simulink model "FullModelAddANN_Final_ANN_revised"  (R2024b)
settings: Solver=ode4  StartTime=0.0  StopTime=40  FixedStep=1e-5  RelTol=1e-3
values from neighbouring files (symbols this model uses):
  Dp = 2.506338228783948e3    (= 2506.33822878)    [FullModelAddANNm_Final.m]    (also in main_opal_ann_control.m)
  Dq = 1.033099625954584    (= 1.03309962595)    [FullModelAddANNm_Final.m]    (also in main_opal_ann_control.m)
  Kp = 0.006383815167581    (= 0.00638381516758)    [FullModelAddANNm_Final.m]    (also in main_opal_ann_control.m)
  Kq = 0.076670166944346    (= 0.0766701669443)    [FullModelAddANNm_Final.m]    (also in main_opal_ann_control.m)
undefined symbols (not defined in the file or in its folder): Filter, Ls, params
libraries: neural x88, spsCurrentMeasurementLib x6, spsParallelRLCBranchLib x6, spsIGBTDiodeLib x6, spsMeanLib x6, spsSeriesRLCBranchLib x6, simulink x4, spsVoltageMeasurementLib x4, spsVariableInductorLib x3, spsVariableResistorLib x3, spsDCVoltageSourceLib x1, spsThreePhaseSourceLib x1
(part 1 of 11)
settings Model: SimulationMode=accelerator  Creator=Admin  LastModifiedBy=ACER
settings DataIOCC: SaveOutput=off  DSMLogging=off  SaveTime=off  ReturnWorkspaceOutputs=off
settings OptimizationCC: EfficientMapNaN2IntZero=off  AccelVerboseBuild=on
settings DebuggingCC: SignalInfNanChecking=error  CheckMatrixSingularityMsg=error  UnconnectedInputMsg=warning  UnconnectedOutputMsg=warning  UnconnectedLineMsg=warning
settings HardwareCC: TargetBitPerPointer=64  TargetBitPerSizeT=64  TargetBitPerPtrDiffT=64  TargetLongLongMode=on  TargetIntDivRoundTo=Zero  TargetEndianess=LittleEndian  TargetWordSize=64  TargetHWDeviceType=MATLAB Host  ProdEqTarget=off
settings ModelReferenceCC: EnableRefExpFcnMdlSchedulingChecks=on
settings SFSimCC: CustomCodeUndefinedFunction=UseInterfaceOnly
settings RTWCC: GPUComputeCapability=3.5
settings CodeAppCC: MaxIdLength=128
settings GRTTargetCC: TargetLangStandard=C89/C90 (ANSI)  CombineOutputUpdateFcns=off  GRTInterface=on

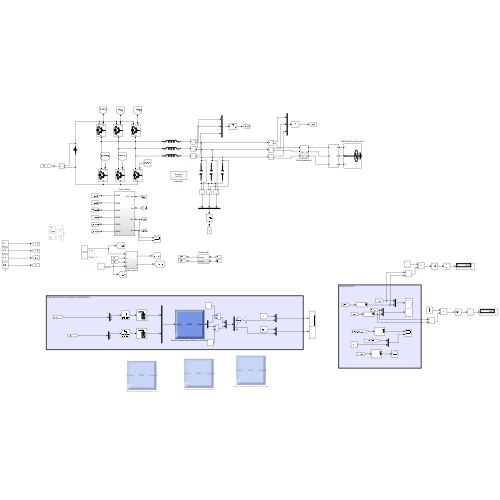
[thumbnail: Simulink's stored preview of the top-level diagram]
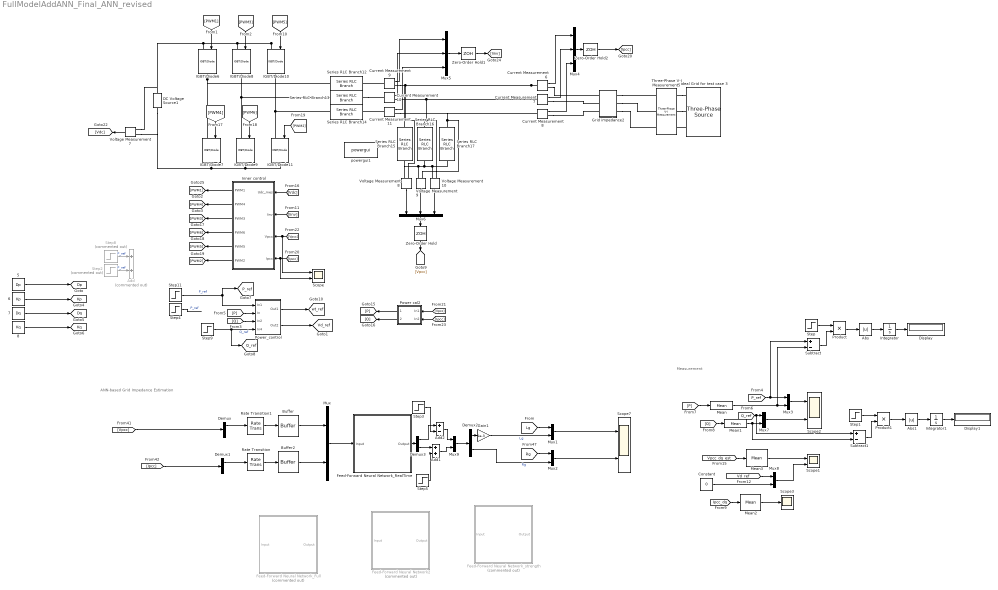
== system FullModelAddANN_Final_ANN_revised ==
  note: Measurement
  note: ANN-based Grid Impedance Estimation
  5 : Constant  Value=Dp
  6 : Constant  Value=Kp
  7 : Constant  Value=Dq
  8 : Constant  Value=Kq
  Abs : Abs  SaturateOnIntegerOverflow=off
  Abs1 : Abs  SaturateOnIntegerOverflow=off
  Add : Sum  Commented=on
  Add1 : Sum
  Add2 : Sum  Inputs=+-
  Buffer : Buffer  N=100  OutputFrames=off
  Buffer2 : Buffer  N=100  OutputFrames=off
  Constant : Constant  Value=0
  Current Measurement{6..11} (6 alike) : spsCurrentMeasurementLib/Current Measurement  PhasorSimulation=off  OutputType=Complex  PSBequivalent=0
  DC Voltage Source1 : spsDCVoltageSourceLib/DC Voltage Source  Amplitude=params.Vdc  Measurements=None
  Demux : Demux  Outputs=3
  Demux1 : Demux  Outputs=3
  Demux2 : Demux  Outputs=2
  Demux3 : Demux  Outputs=2
  Display : Display
  Display1 : Display
  Feed-Forward Neural Network2 : Subsystem  Commented=on
      mask help: Feed-Forward Neural Network
      mask Display: e = 0.06;c1 = [120 150 230]/255;c2 = ([120 150 230]+0)/383;c3 = ([120 150 230]+128)/383;patch([0 1 1 0],[0 0 1 1],c1);patch([0 1 1 1-e 1-e 0+e],[0 0 1 1-e 0+e 0+e],c2);patch([0 0 1 1-e 0+e 0+e],[0 1 1 1-e 1-e 0+e],c3);plot([0 1 1 0 0],[0 0 1 1 0]);fprintf('NNET');port_label('input',1,' Input');port_label('output',1,'Output ');
  Feed-Forward Neural Network_Full : Subsystem  Commented=on
      mask help: Feed-Forward Neural Network
      mask Display: e = 0.06;c1 = [120 150 230]/255;c2 = ([120 150 230]+0)/383;c3 = ([120 150 230]+128)/383;patch([0 1 1 0],[0 0 1 1],c1);patch([0 1 1 1-e 1-e 0+e],[0 0 1 1-e 0+e 0+e],c2);patch([0 0 1 1-e 0+e 0+e],[0 1 1 1-e 1-e 0+e],c3);plot([0 1 1 0 0],[0 0 1 1 0]);fprintf('NNET');port_label('input',1,' Input');port_label('output',1,'Output ');
  Feed-Forward Neural Network_RealTime : Subsystem
      mask help: Feed-Forward Neural Network
      mask Display: e = 0.06;c1 = [120 150 230]/255;c2 = ([120 150 230]+0)/383;c3 = ([120 150 230]+128)/383;patch([0 1 1 0],[0 0 1 1],c1);patch([0 1 1 1-e 1-e 0+e],[0 0 1 1-e 0+e 0+e],c2);patch([0 0 1 1-e 0+e 0+e],[0 1 1 1-e 1-e 0+e],c3);plot([0 1 1 0 0],[0 0 1 1 0]);fprintf('NNET');port_label('input',1,' Input');port_label('output',1,'Output ');
  Feed-Forward Neural Network_strength : Subsystem  Commented=on
      mask help: Feed-Forward Neural Network
      mask Display: e = 0.06;c1 = [120 150 230]/255;c2 = ([120 150 230]+0)/383;c3 = ([120 150 230]+128)/383;patch([0 1 1 0],[0 0 1 1],c1);patch([0 1 1 1-e 1-e 0+e],[0 0 1 1-e 0+e 0+e],c2);patch([0 0 1 1-e 0+e 0+e],[0 1 1 1-e 1-e 0+e],c3);plot([0 1 1 0 0],[0 0 1 1 0]);fprintf('NNET');port_label('input',1,' Input');port_label('output',1,'Output ');
  Gain1 : Gain  Gain=1e-3
  Grid impedance2 : Subsystem
  IGBT/Diode{6..11} (6 alike) : spsIGBTDiodeLib/IGBT//Diode  Ron=1e-3  Rs=1e5  Cs=inf  Measurements=off
  Ideal Grid for test case 3 : spsThreePhaseSourceLib/Three-Phase Source  InternalConnection=Yg  VoltagePhases=off  Voltage=params.Vj*sqrt(3)  PhaseAngle=0  Voltage_phases=[25e3 25e3 25e3]/sqrt(3)  PhaseAngles_phases=[0 -120 +120]  Frequency=params.f0  NonIdealSource=off  SpecifyImpedance=on  Resistance=0.8929  Inductance=16.58e-3  ShortCircuitLevel=params.SCR*params.S_rated  BaseVoltage=params.Vll_rms  XRratio=params.XR  BusType=swing  Pref=1e3  Qref=0  Prefabc=[10e3, 10e3, 10e3]  Qrefabc=[0, 0, 0]  Qmin=-inf  Qmax=inf
  Inner control : Subsystem
  Integrator : Integrator
  Integrator1 : Integrator
  Mean : spsMeanLib/Mean  Freq=50  Vinit=0  Ts=0
  Mean1 : spsMeanLib/Mean  Freq=50  Vinit=0  Ts=0
  Mean2 : spsMeanLib/Mean  Freq=60  Vinit=0  Ts=0
  Mean3 : spsMeanLib/Mean  Freq=60  Vinit=0  Ts=0
  Mux{,1..3,7..9} (7 alike) : Mux  Inputs=2
  Mux4 : Mux  Inputs=3
  Mux5 : Mux  Inputs=3
  Mux6 : Mux  Inputs=3
  Power cal2 : Subsystem
  Power_control : Subsystem
  Product : Product
  Product1 : Product
  Rate Transition : RateTransition  OutPortSampleTimeMultiple=2e-4  OutPortSampleTime=2e-4
  Rate Transition1 : RateTransition  OutPortSampleTimeMultiple=4  OutPortSampleTime=2e-4
  Scope{,1..2,7} (4 alike) : Scope  NumInputPorts=2
  Scope3 : Scope
  Series RLC Branch12 : spsSeriesRLCBranchLib/Series RLC Branch  LConnTagsString=__new0  RConnTagsString=__new0  BranchType=L  Resistance=Filter.Rs_1  Inductance=params.Filter.Ls_1  SetiL0=off  InitialCurrent=1  Capacitance=1e-6  Setx0=off  InitialVoltage=0  Measurements=None
  Series RLC Branch13 : spsSeriesRLCBranchLib/Series RLC Branch  LConnTagsString=__new0  RConnTagsString=__new0  BranchType=L  Resistance=Filter.Rs_1  Inductance=params.Filter.Ls_1  SetiL0=off  InitialCurrent=1  Capacitance=1e-6  Setx0=off  InitialVoltage=0  Measurements=None
  Series RLC Branch14 : spsSeriesRLCBranchLib/Series RLC Branch  LConnTagsString=__new0  RConnTagsString=__new0  BranchType=L  Resistance=Filter.Rs_1  Inductance=params.Filter.Ls_1  SetiL0=off  InitialCurrent=1  Capacitance=1e-6  Setx0=off  InitialVoltage=0  Measurements=None
  Series RLC Branch15 : spsSeriesRLCBranchLib/Series RLC Branch  LConnTagsString=__new0  RConnTagsString=__new0  BranchType=C  Resistance=1  Inductance=Ls  SetiL0=off  InitialCurrent=0  Capacitance=params.Filter.Cs  Setx0=off  InitialVoltage=0  Measurements=None
  Series RLC Branch16 : spsSeriesRLCBranchLib/Series RLC Branch  LConnTagsString=__new0  RConnTagsString=__new0  BranchType=C  Resistance=1  Inductance=Ls  SetiL0=off  InitialCurrent=0  Capacitance=params.Filter.Cs  Setx0=off  InitialVoltage=0  Measurements=None
  Series RLC Branch17 : spsSeriesRLCBranchLib/Series RLC Branch  LConnTagsString=__new0  RConnTagsString=__new0  BranchType=C  Resistance=1  Inductance=Ls  SetiL0=off  InitialCurrent=0  Capacitance=params.Filter.Cs  Setx0=off  InitialVoltage=0  Measurements=None
  Step : Step  Time=20  SampleTime=0
  Step1 : Step  Time=20  SampleTime=0
  Step11 : Step  Time=30  Before=3.5e3  After=4e3  SampleTime=0
  Step2 : Step  Commented=on  Time=70  After=0.5e3  SampleTime=0
  Step3 : Step  Time=20  After=4.08  SampleTime=0
  Step4 : Step  Time=70  After=0.5e3  SampleTime=0
  Step5 : Step  Time=20  SampleTime=0
  Step8 : Step  Commented=on  Time=50  Before=4e3  After=3.5e3  SampleTime=0
  Step9 : Step  Time=90  Before=params.Qref  After=params.Qref-0.5e3  SampleTime=0
  Subtract : Sum  Inputs=+-
  Subtract1 : Sum  Inputs=+-
  Three-Phase V-I Measurement5 : spsThreePhaseVIMeasurementLib/Three-Phase V-I Measurement  VoltageMeasurement=no  SetLabelV=off  LabelV=Vabc  Vpu=off  VpuLL=off  CurrentMeasurement=no  SetLabelI=off  LabelI=Iabc  Ipu=off  Pbase=100e6  Vbase=500e3  OutputType=Complex  PhasorSimulation=off  PSBequivalent=0
  Voltage Measurement{7..10} (4 alike) : spsVoltageMeasurementLib/Voltage Measurement  PhasorSimulation=off  OutputType=Complex  PSBequivalent=0
  Zero-Order Hold : ZeroOrderHold  SampleTime=5e-5
  Zero-Order Hold1 : ZeroOrderHold  SampleTime=5e-5
  Zero-Order Hold2 : ZeroOrderHold  SampleTime=5e-5
  powergui1 : sps_lib/powergui  Priority=1  SimulationMode=Discrete  SampleTime=1e-5  frequency=60  Iterations=50  frequencyindice=0  Pbase=100e6  ErrMax=1e-4  UnitsV=kV  UnitsW=MW  buscounter=0  FunctionMessages=off  echomessages=off  EnableUseOfTLC=off  CurrentSourceSwitches=off  DisableSnubberDevices=off  DisableRonSwitches=off  DisableVfSwitches=off  DisplayEquations=off  AutomaticDiscreteSolvers=on  SolverType=Tustin/Backward Euler (TBE)  Interpol=off  ExternalGateDelay=off  methode=off  Ts=100  x0status=blocks  SPID=on  SwTol=0  HookPort=off  NonlinearTolerance=0  nMaxIteration=15  ContinueOnMaxIteration=off  RestoreLinks=warning  ResistiveCurrentMeasurement=off  Frange=[0:2:500]  Ylog=off  Xlog=on  ShowGrid=off  save=off  variable=ZData  structure=0  ZoomFFT=off  StartTime=0.0  cycles=1  DisplayStyle=1  fundamental=60  FreqAxis=off  MaxFrequency=1000  frequencyindicesteady=1  RmsSteady=1  display=off
  tag scope: Dp=global, Dq=global, Kp=global, Kq=global, P_ref=global, Q_ref=global, Vd_ref=global, wt_ref=global
  wires:
  Step8/1 -> Add/1  "P_ref"
  Step2/1 -> Add/2  "P_ref"
  [Iinv] -> Inner control/2(Iinv)
  Inner control/1(PWM1) -> [PWM1]
  Inner control/4("PWM6 ") -> [PWM6]
  Inner control/6(PWM2) -> [PWM2]
  Voltage Measurement7/1 -> [Vdc]
  Inner control/5(PWM5) -> [PWM5]
  Voltage Measurement9/1 -> Mux6/2
  Mux5/1 -> Zero-Order Hold1/1
  [PWM6] -> IGBT/Diode9/1
  [PWM1] -> IGBT/Diode6/1
  [Ipcc] -> Scope/2, Inner control/4(Ipcc)
  [Vdc] -> Inner control/1(Udc_mes)
  [Vpcc] -> Scope/1, Inner control/3(Vpcc)
  Inner control/3(PWM3) -> [PWM3]
  Inner control/2("PWM4 ") -> [PWM4]
  Current Measurement11/1 -> Mux5/3
  Voltage Measurement10/1 -> Mux6/3
  [PWM2] -> IGBT/Diode11/1
  Mux4/1 -> Zero-Order Hold2/1
  [PWM4] -> IGBT/Diode7/1
  Mux6/1 -> Zero-Order Hold/1
  [PWM5] -> IGBT/Diode10/1
  Current Measurement8/1 -> Mux4/3
  Voltage Measurement8/1 -> Mux6/1
  Current Measurement9/1 -> Mux5/1
  Current Measurement7/1 -> Mux4/2
  Current Measurement6/1 -> Mux4/1
  Current Measurement10/1 -> Mux5/2
  [PWM3] -> IGBT/Diode8/1
  Power cal2/2(deltay2) -> [Q]
  Power cal2/1(deltay1) -> [P]
  [Vpcc] -> Power cal2/1(In1)
  [Ipcc] -> Power cal2/2(In2)
  Zero-Order Hold/1 -> [Vpcc]
  Zero-Order Hold1/1 -> [Iinv]
  Zero-Order Hold2/1 -> [Ipcc]
  5/1 -> [Dp]
  6/1 -> [Kp]
  7/1 -> [Dq]
  8/1 -> [Kq]
  Rate Transition1/1 -> Buffer/1
  Demux1/1 -> Rate Transition/1
  Demux/1 -> Rate Transition1/1
  Rate Transition/1 -> Buffer2/1
  Buffer2/1 -> Mux/2
  Buffer/1 -> Mux/1
  Mux/1 -> Feed-Forward Neural Network_RealTime/1(Input)
  Demux2/1 -> Gain1/1
  [P] -> Power_control/2(In)
  [Q] -> Power_control/3(In2)
  Power_control/1(Out1) -> [wt_ref]
  Power_control/2(Out2) -> [Vd_ref]
  [Lg] -> Mux1/1
  Gain1/1 -> Mux1/2  "Lg"
  [Rg] -> Mux2/1
  Demux2/2 -> Mux2/2  "Rg"
  Mux1/1 -> Scope7/1
  Mux2/1 -> Scope7/2
  [Vpcc] -> Demux/1
  [Ipcc] -> Demux1/1
  [Q] -> Mean1/1
  [P] -> Mean/1
  [Q_ref] -> Subtract1/1, Mux7/1
  Mux7/1 -> Scope2/2
  [P_ref] -> Subtract/1, Mux3/1
  Mux3/1 -> Scope2/1
  Mean1/1 -> Subtract1/2, Mux7/2
  Mean/1 -> Subtract/2, Mux3/2
  Mux8/1 -> Scope1/2
  Mean2/1 -> Scope3/1
  Constant/1 -> Mux8/2
  Mean3/1 -> Scope1/1
  [Vpcc_dq_est] -> Mean3/1
  [Ipcc_dq] -> Mean2/1
  [Vd_ref] -> Mux8/1
  Step4/1 -> ?  "P_ref"
  Step11/1 -> Power_control/1(In1), [P_ref]  "P_ref"
  Step9/1 -> [Q_ref], Power_control/4(In4)  "Q_ref"
  Abs/1 -> Integrator/1
  Integrator/1 -> Display/1
  Integrator1/1 -> Display1/1
  Abs1/1 -> Integrator1/1
  Step/1 -> Product/1
  Subtract/1 -> Product/2
  Product/1 -> Abs/1
  Step1/1 -> Product1/1
  Subtract1/1 -> Product1/2
  Product1/1 -> Abs1/1
  Feed-Forward Neural Network_RealTime/1(Output) -> Demux3/1
  Mux9/1 -> Demux2/1
  Demux3/1 -> Add2/1
  Add2/1 -> Mux9/1
  Demux3/2 -> Add1/1
  Add1/1 -> Mux9/2
  Step5/1 -> Add1/2
  Step3/1 -> Add2/2
  connections:
  Series RLC Branch14/LConn1 -- IGBT/Diode10/RConn1 -- IGBT/Diode11/LConn1
  Series RLC Branch17/LConn1 -- Current Measurement11/RConn1 -- Current Measurement8/LConn1 -- Voltage Measurement10/LConn1
  IGBT/Diode6/RConn1 -- Series RLC Branch12/LConn1 -- IGBT/Diode7/LConn1
  Voltage Measurement10/LConn2 -- Series RLC Branch17/RConn1 -- Voltage Measurement8/LConn2 -- Series RLC Branch15/RConn1 -- Voltage Measurement9/LConn2 -- Series RLC Branch16/RConn1
  Current Measurement6/LConn1 -- Series RLC Branch15/LConn1 -- Voltage Measurement8/LConn1 -- Current Measurement9/RConn1
  IGBT/Diode10/LConn1 -- DC Voltage Source1/RConn1 -- Voltage Measurement7/LConn1 -- IGBT/Diode6/LConn1 -- IGBT/Diode8/LConn1
  IGBT/Diode7/RConn1 -- IGBT/Diode11/RConn1 -- IGBT/Diode9/RConn1 -- Voltage Measurement7/LConn2 -- DC Voltage Source1/LConn1
  Series RLC Branch13/LConn1 -- IGBT/Diode8/RConn1 -- IGBT/Diode9/LConn1
  Current Measurement7/LConn1 -- Current Measurement10/RConn1 -- Series RLC Branch16/LConn1 -- Voltage Measurement9/LConn1
  Current Measurement7/RConn1 -- Grid impedance2/LConn2
  Current Measurement11/LConn1 -- Series RLC Branch14/RConn1
  Current Measurement8/RConn1 -- Grid impedance2/LConn3
  Series RLC Branch13/RConn1 -- Current Measurement10/LConn1
  Current Measurement9/LConn1 -- Series RLC Branch12/RConn1
  Current Measurement6/RConn1 -- Grid impedance2/LConn1
  Grid impedance2/RConn1 -- Three-Phase V-I Measurement5/RConn3
  Three-Phase V-I Measurement5/LConn2 -- Ideal Grid for test case 3/RConn2
  Three-Phase V-I Measurement5/LConn3 -- Ideal Grid for test case 3/RConn3
  Grid impedance2/RConn2 -- Three-Phase V-I Measurement5/RConn2
  Ideal Grid for test case 3/RConn1 -- Three-Phase V-I Measurement5/LConn1
  Grid impedance2/RConn3 -- Three-Phase V-I Measurement5/RConn1

== system FullModelAddANN_Final_ANN_revised/Feed-Forward Neural Network2 ==
  Input : Inport  PortDimensions=200
      mask Display: e = 0.06;c1 = [120 230 180]/255;c2 = ([120 230 180]+0)/(256+128);c3 = ([120 230 180]+128)/(256+128);patch([0 1 1 0],[0 0 1 1],c1);patch([0 1 1 1-e 1-e 0+e],[0 0 1 1-e 0+e 0+e],c2);patch([0 0 1 1-e 0+e 0+e],[0 1 1 1-e 1-e 0+e],c3);plot([0 1 1 0 0],[0 0 1 1 0]);
  Layer 1 : Subsystem
      mask Display: e = 0.06;c1 = [120 150 230]/255;c2 = ([120 150 230]+0)/383;c3 = ([120 150 230]+128)/383;patch([0 1 1 0],[0 0 1 1],c1);patch([0 1 1 1-e 1-e 0+e],[0 0 1 1-e 0+e 0+e],c2);patch([0 0 1 1-e 0+e 0+e],[0 1 1 1-e 1-e 0+e],c3);plot([0 1 1 0 0],[0 0 1 1 0]);
  Layer 2 : Subsystem
      mask Display: e = 0.06;c1 = [120 150 230]/255;c2 = ([120 150 230]+0)/383;c3 = ([120 150 230]+128)/383;patch([0 1 1 0],[0 0 1 1],c1);patch([0 1 1 1-e 1-e 0+e],[0 0 1 1-e 0+e 0+e],c2);patch([0 0 1 1-e 0+e 0+e],[0 1 1 1-e 1-e 0+e],c3);plot([0 1 1 0 0],[0 0 1 1 0]);
  Process Input 1 : Subsystem
      mask Display: e = 0.06;c1 = [120 150 230]/255;c2 = ([120 150 230]+0)/383;c3 = ([120 150 230]+128)/383;patch([0 1 1 0],[0 0 1 1],c1);patch([0 1 1 1-e 1-e 0+e],[0 0 1 1-e 0+e 0+e],c2);patch([0 0 1 1-e 0+e 0+e],[0 1 1 1-e 1-e 0+e],c3);plot([0 1 1 0 0],[0 0 1 1 0]);
  Process Output 1 : Subsystem
      mask Display: e = 0.06;c1 = [120 150 230]/255;c2 = ([120 150 230]+0)/383;c3 = ([120 150 230]+128)/383;patch([0 1 1 0],[0 0 1 1],c1);patch([0 1 1 1-e 1-e 0+e],[0 0 1 1-e 0+e 0+e],c2);patch([0 0 1 1-e 0+e 0+e],[0 1 1 1-e 1-e 0+e],c3);plot([0 1 1 0 0],[0 0 1 1 0]);
  Output : Outport  InitialOutput=[0;0]
      mask Display: e = 0.06;c1 = [120 230 180]/255;c2 = ([120 230 180]+0)/(256+128);c3 = ([120 230 180]+128)/(256+128);patch([0 1 1 0],[0 0 1 1],c1);patch([0 1 1 1-e 1-e 0+e],[0 0 1 1-e 0+e 0+e],c2);patch([0 0 1 1-e 0+e 0+e],[0 1 1 1-e 1-e 0+e],c3);plot([0 1 1 0 0],[0 0 1 1 0]);
  wires:
  Input/1 -> Process Input 1/1(x)
  Process Output 1/1(y) -> Output/1
  Process Input 1/1(p) -> Layer 1/1("p{1}")
  Layer 1/1("a{1}") -> [feedback1]
  [feedback1] -> Layer 2/1("a{1} ")
  Layer 2/1("a{2}") -> Process Output 1/1(a)

== system FullModelAddANN_Final_ANN_revised/Feed-Forward Neural Network_Full ==
  Input : Inport  PortDimensions=200
      mask Display: e = 0.06;c1 = [120 230 180]/255;c2 = ([120 230 180]+0)/(256+128);c3 = ([120 230 180]+128)/(256+128);patch([0 1 1 0],[0 0 1 1],c1);patch([0 1 1 1-e 1-e 0+e],[0 0 1 1-e 0+e 0+e],c2);patch([0 0 1 1-e 0+e 0+e],[0 1 1 1-e 1-e 0+e],c3);plot([0 1 1 0 0],[0 0 1 1 0]);
  Layer 1 : Subsystem
      mask Display: e = 0.06;c1 = [120 150 230]/255;c2 = ([120 150 230]+0)/383;c3 = ([120 150 230]+128)/383;patch([0 1 1 0],[0 0 1 1],c1);patch([0 1 1 1-e 1-e 0+e],[0 0 1 1-e 0+e 0+e],c2);patch([0 0 1 1-e 0+e 0+e],[0 1 1 1-e 1-e 0+e],c3);plot([0 1 1 0 0],[0 0 1 1 0]);
  Layer 2 : Subsystem
      mask Display: e = 0.06;c1 = [120 150 230]/255;c2 = ([120 150 230]+0)/383;c3 = ([120 150 230]+128)/383;patch([0 1 1 0],[0 0 1 1],c1);patch([0 1 1 1-e 1-e 0+e],[0 0 1 1-e 0+e 0+e],c2);patch([0 0 1 1-e 0+e 0+e],[0 1 1 1-e 1-e 0+e],c3);plot([0 1 1 0 0],[0 0 1 1 0]);
  Process Input 1 : Subsystem
      mask Display: e = 0.06;c1 = [120 150 230]/255;c2 = ([120 150 230]+0)/383;c3 = ([120 150 230]+128)/383;patch([0 1 1 0],[0 0 1 1],c1);patch([0 1 1 1-e 1-e 0+e],[0 0 1 1-e 0+e 0+e],c2);patch([0 0 1 1-e 0+e 0+e],[0 1 1 1-e 1-e 0+e],c3);plot([0 1 1 0 0],[0 0 1 1 0]);
  Process Output 1 : Subsystem
      mask Display: e = 0.06;c1 = [120 150 230]/255;c2 = ([120 150 230]+0)/383;c3 = ([120 150 230]+128)/383;patch([0 1 1 0],[0 0 1 1],c1);patch([0 1 1 1-e 1-e 0+e],[0 0 1 1-e 0+e 0+e],c2);patch([0 0 1 1-e 0+e 0+e],[0 1 1 1-e 1-e 0+e],c3);plot([0 1 1 0 0],[0 0 1 1 0]);
  Output : Outport  InitialOutput=[0;0]
      mask Display: e = 0.06;c1 = [120 230 180]/255;c2 = ([120 230 180]+0)/(256+128);c3 = ([120 230 180]+128)/(256+128);patch([0 1 1 0],[0 0 1 1],c1);patch([0 1 1 1-e 1-e 0+e],[0 0 1 1-e 0+e 0+e],c2);patch([0 0 1 1-e 0+e 0+e],[0 1 1 1-e 1-e 0+e],c3);plot([0 1 1 0 0],[0 0 1 1 0]);
  wires:
  Input/1 -> Process Input 1/1(x)
  Process Output 1/1(y) -> Output/1
  Process Input 1/1(p) -> Layer 1/1("p{1}")
  Layer 1/1("a{1}") -> [feedback1]
  [feedback1] -> Layer 2/1("a{1} ")
  Layer 2/1("a{2}") -> Process Output 1/1(a)

== system FullModelAddANN_Final_ANN_revised/Feed-Forward Neural Network_RealTime ==
  Input : Inport  PortDimensions=200
      mask Display: e = 0.06;c1 = [120 230 180]/255;c2 = ([120 230 180]+0)/(256+128);c3 = ([120 230 180]+128)/(256+128);patch([0 1 1 0],[0 0 1 1],c1);patch([0 1 1 1-e 1-e 0+e],[0 0 1 1-e 0+e 0+e],c2);patch([0 0 1 1-e 0+e 0+e],[0 1 1 1-e 1-e 0+e],c3);plot([0 1 1 0 0],[0 0 1 1 0]);
  Layer 1 : Subsystem
      mask Display: e = 0.06;c1 = [120 150 230]/255;c2 = ([120 150 230]+0)/383;c3 = ([120 150 230]+128)/383;patch([0 1 1 0],[0 0 1 1],c1);patch([0 1 1 1-e 1-e 0+e],[0 0 1 1-e 0+e 0+e],c2);patch([0 0 1 1-e 0+e 0+e],[0 1 1 1-e 1-e 0+e],c3);plot([0 1 1 0 0],[0 0 1 1 0]);
  Layer 2 : Subsystem
      mask Display: e = 0.06;c1 = [120 150 230]/255;c2 = ([120 150 230]+0)/383;c3 = ([120 150 230]+128)/383;patch([0 1 1 0],[0 0 1 1],c1);patch([0 1 1 1-e 1-e 0+e],[0 0 1 1-e 0+e 0+e],c2);patch([0 0 1 1-e 0+e 0+e],[0 1 1 1-e 1-e 0+e],c3);plot([0 1 1 0 0],[0 0 1 1 0]);
  Process Input 1 : Subsystem
      mask Display: e = 0.06;c1 = [120 150 230]/255;c2 = ([120 150 230]+0)/383;c3 = ([120 150 230]+128)/383;patch([0 1 1 0],[0 0 1 1],c1);patch([0 1 1 1-e 1-e 0+e],[0 0 1 1-e 0+e 0+e],c2);patch([0 0 1 1-e 0+e 0+e],[0 1 1 1-e 1-e 0+e],c3);plot([0 1 1 0 0],[0 0 1 1 0]);
  Process Output 1 : Subsystem
      mask Display: e = 0.06;c1 = [120 150 230]/255;c2 = ([120 150 230]+0)/383;c3 = ([120 150 230]+128)/383;patch([0 1 1 0],[0 0 1 1],c1);patch([0 1 1 1-e 1-e 0+e],[0 0 1 1-e 0+e 0+e],c2);patch([0 0 1 1-e 0+e 0+e],[0 1 1 1-e 1-e 0+e],c3);plot([0 1 1 0 0],[0 0 1 1 0]);
  Output : Outport  InitialOutput=[0;0]
      mask Display: e = 0.06;c1 = [120 230 180]/255;c2 = ([120 230 180]+0)/(256+128);c3 = ([120 230 180]+128)/(256+128);patch([0 1 1 0],[0 0 1 1],c1);patch([0 1 1 1-e 1-e 0+e],[0 0 1 1-e 0+e 0+e],c2);patch([0 0 1 1-e 0+e 0+e],[0 1 1 1-e 1-e 0+e],c3);plot([0 1 1 0 0],[0 0 1 1 0]);
  wires:
  Input/1 -> Process Input 1/1(x)
  Process Output 1/1(y) -> Output/1
  Process Input 1/1(p) -> Layer 1/1("p{1}")
  Layer 1/1("a{1}") -> [feedback1]
  [feedback1] -> Layer 2/1("a{1} ")
  Layer 2/1("a{2}") -> Process Output 1/1(a)

== system FullModelAddANN_Final_ANN_revised/Feed-Forward Neural Network_strength ==
  Input : Inport  PortDimensions=200
      mask Display: e = 0.06;c1 = [120 230 180]/255;c2 = ([120 230 180]+0)/(256+128);c3 = ([120 230 180]+128)/(256+128);patch([0 1 1 0],[0 0 1 1],c1);patch([0 1 1 1-e 1-e 0+e],[0 0 1 1-e 0+e 0+e],c2);patch([0 0 1 1-e 0+e 0+e],[0 1 1 1-e 1-e 0+e],c3);plot([0 1 1 0 0],[0 0 1 1 0]);
  Layer 1 : Subsystem
      mask Display: e = 0.06;c1 = [120 150 230]/255;c2 = ([120 150 230]+0)/383;c3 = ([120 150 230]+128)/383;patch([0 1 1 0],[0 0 1 1],c1);patch([0 1 1 1-e 1-e 0+e],[0 0 1 1-e 0+e 0+e],c2);patch([0 0 1 1-e 0+e 0+e],[0 1 1 1-e 1-e 0+e],c3);plot([0 1 1 0 0],[0 0 1 1 0]);
  Layer 2 : Subsystem
      mask Display: e = 0.06;c1 = [120 150 230]/255;c2 = ([120 150 230]+0)/383;c3 = ([120 150 230]+128)/383;patch([0 1 1 0],[0 0 1 1],c1);patch([0 1 1 1-e 1-e 0+e],[0 0 1 1-e 0+e 0+e],c2);patch([0 0 1 1-e 0+e 0+e],[0 1 1 1-e 1-e 0+e],c3);plot([0 1 1 0 0],[0 0 1 1 0]);
  Process Input 1 : Subsystem
      mask Display: e = 0.06;c1 = [120 150 230]/255;c2 = ([120 150 230]+0)/383;c3 = ([120 150 230]+128)/383;patch([0 1 1 0],[0 0 1 1],c1);patch([0 1 1 1-e 1-e 0+e],[0 0 1 1-e 0+e 0+e],c2);patch([0 0 1 1-e 0+e 0+e],[0 1 1 1-e 1-e 0+e],c3);plot([0 1 1 0 0],[0 0 1 1 0]);
  Process Output 1 : Subsystem
      mask Display: e = 0.06;c1 = [120 150 230]/255;c2 = ([120 150 230]+0)/383;c3 = ([120 150 230]+128)/383;patch([0 1 1 0],[0 0 1 1],c1);patch([0 1 1 1-e 1-e 0+e],[0 0 1 1-e 0+e 0+e],c2);patch([0 0 1 1-e 0+e 0+e],[0 1 1 1-e 1-e 0+e],c3);plot([0 1 1 0 0],[0 0 1 1 0]);
  Output : Outport  InitialOutput=[0;0]
      mask Display: e = 0.06;c1 = [120 230 180]/255;c2 = ([120 230 180]+0)/(256+128);c3 = ([120 230 180]+128)/(256+128);patch([0 1 1 0],[0 0 1 1],c1);patch([0 1 1 1-e 1-e 0+e],[0 0 1 1-e 0+e 0+e],c2);patch([0 0 1 1-e 0+e 0+e],[0 1 1 1-e 1-e 0+e],c3);plot([0 1 1 0 0],[0 0 1 1 0]);
  wires:
  Input/1 -> Process Input 1/1(x)
  Process Output 1/1(y) -> Output/1
  Process Input 1/1(p) -> Layer 1/1("p{1}")
  Layer 1/1("a{1}") -> [feedback1]
  [feedback1] -> Layer 2/1("a{1} ")
  Layer 2/1("a{2}") -> Process Output 1/1(a)

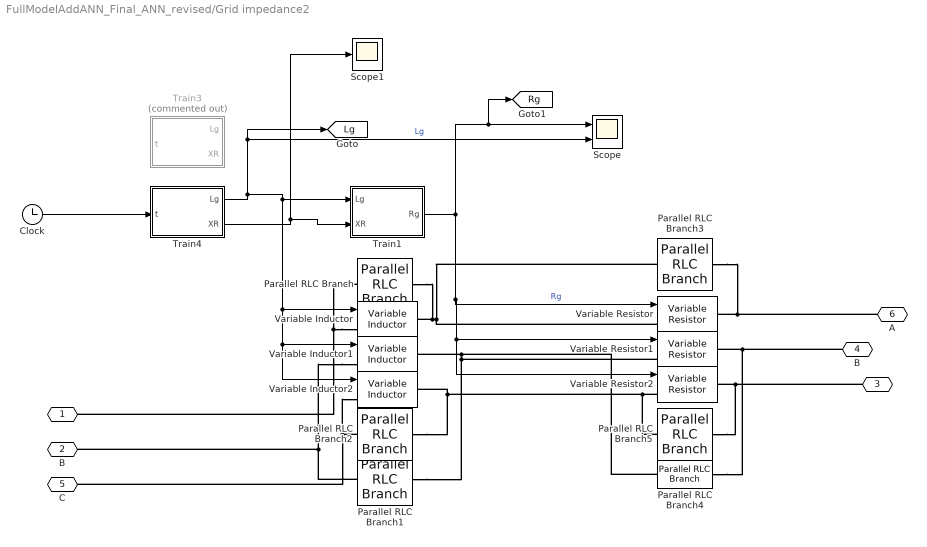
== system FullModelAddANN_Final_ANN_revised/Grid impedance2 ==
  Clock : Clock
      settings: Decimation=150
  Parallel RLC Branch{,1..5} (6 alike) : spsParallelRLCBranchLib/Parallel RLC Branch  LConnTagsString=a  RConnTagsString=__new0  BranchType=R  Resistance=1e6  Inductance=1e-3  SetiL0=off  InitialCurrent=0  Capacitance=1e-6  Setx0=off  InitialVoltage=0  Measurements=None
  Scope : Scope  NumInputPorts=2
  Scope1 : Scope
  Train1 : MATLAB Function  TreatAsAtomicUnit=on
  Train3 : MATLAB Function  Commented=on  TreatAsAtomicUnit=on
  Train4 : MATLAB Function  TreatAsAtomicUnit=on
  Variable Inductor : spsVariableInductorLib/Variable Inductor  methode=Backward Euler  Labsmin=1e-6  Initialize=off  iL0=0  L0=1e-3  Vl0=-0.0024759
  Variable Inductor1 : spsVariableInductorLib/Variable Inductor  methode=Backward Euler  Labsmin=1e-6  Initialize=off  iL0=0  L0=1e-3  Vl0=67.3622
  Variable Inductor2 : spsVariableInductorLib/Variable Inductor  methode=Backward Euler  Labsmin=1e-6  Initialize=off  iL0=0  L0=1e-3  Vl0=-67.3597
  Variable Resistor : spsVariableResistorLib/Variable Resistor  Rabsmin=1e-3
  Variable Resistor1 : spsVariableResistorLib/Variable Resistor  Rabsmin=1e-3
  Variable Resistor2 : spsVariableResistorLib/Variable Resistor  Rabsmin=1e-3
  "   " : PMIOPort  Side=Left
  "   B" : PMIOPort  Port=2  Side=Left
  "  " : PMIOPort  Port=3  Side=Right
  "  B" : PMIOPort  Port=4  Side=Right
  "   C" : PMIOPort  Port=5  Side=Left
  "  A" : PMIOPort  Port=6  Side=Right
  tag scope: Lg=global, Rg=global
  wires:
  Train1/1(Rg) -> Scope/1, [Rg], Variable Resistor/1, Variable Resistor1/1, Variable Resistor2/1  "Rg"
  Clock/1 -> Train4/1(t)
  Train4/1(Lg) -> [Lg], Scope/2, Variable Inductor/1, Variable Inductor1/1, Variable Inductor2/1, Train1/1(Lg)  "Lg"
  Train4/2(XR) -> Train1/2(XR), Scope1/1
  connections:
  Variable Resistor1/LConn1 -- Variable Inductor1/RConn1 -- Parallel RLC Branch4/LConn1 -- Parallel RLC Branch1/RConn1
  Variable Resistor2/LConn1 -- Parallel RLC Branch5/LConn1 -- Variable Inductor2/RConn1 -- Parallel RLC Branch2/RConn1
  Variable Resistor1/RConn1 -- Parallel RLC Branch4/RConn1 -- "  B"/RConn1
  Variable Resistor2/RConn1 -- Parallel RLC Branch5/RConn1 -- "  "/RConn1
  Variable Resistor/RConn1 -- Parallel RLC Branch3/RConn1 -- "  A"/RConn1
  Variable Inductor/LConn1 -- "   "/RConn1 -- Parallel RLC Branch/LConn1
  Variable Inductor/RConn1 -- Parallel RLC Branch3/LConn1 -- Variable Resistor/LConn1 -- Parallel RLC Branch/RConn1
  Variable Inductor1/LConn1 -- "   B"/RConn1 -- Parallel RLC Branch1/LConn1
  Variable Inductor2/LConn1 -- "   C"/RConn1 -- Parallel RLC Branch2/LConn1

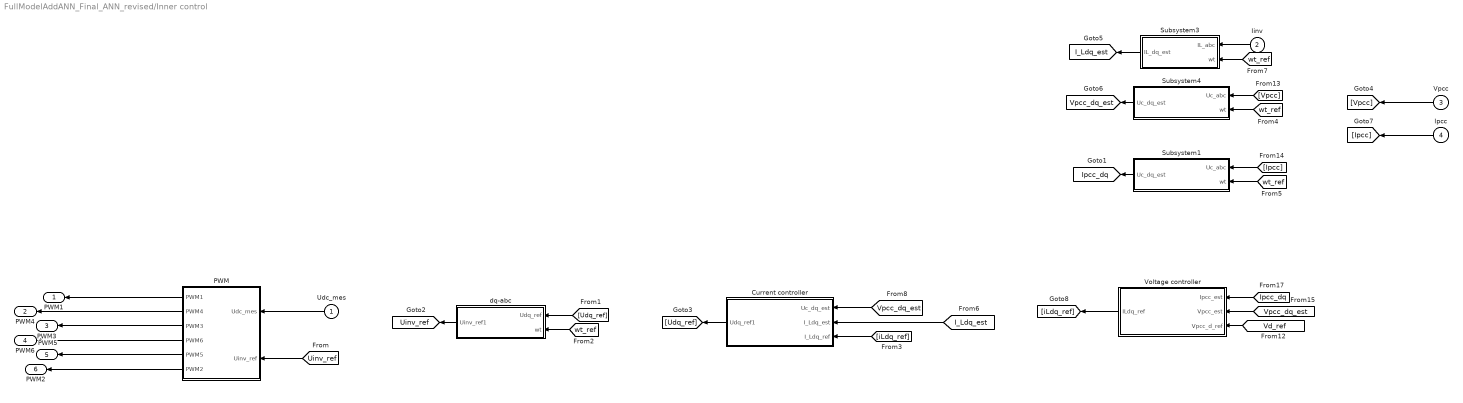
== system FullModelAddANN_Final_ANN_revised/Inner control ==
  Udc_mes : Inport
  Iinv : Inport  Port=2
  Vpcc : Inport  Port=3
  Ipcc : Inport  Port=4
  Current controller : Subsystem
  PWM : Subsystem
  Subsystem1 : Subsystem
  Subsystem3 : Subsystem
  Subsystem4 : Subsystem
  Voltage controller : Subsystem
  dq-abc : Subsystem
  PWM1 : Outport
  "PWM4 " : Outport  Port=2
  PWM3 : Outport  Port=3
  "PWM6 " : Outport  Port=4
  PWM5 : Outport  Port=5
  PWM2 : Outport  Port=6
  tag scope: I_Ldq_est=global, Ipcc_dq=global, Uinv_ref=global, Vpcc_dq_est=global
  wires:
  [Vpcc_dq_est] -> Current controller/1(Uc_dq_est)
  PWM/4("PWM6 ") -> "PWM6 "/1
  Udc_mes/1 -> PWM/1(Udc_mes)
  [I_Ldq_est] -> Current controller/2(I_Ldq_est)
  Subsystem4/1(Uc_dq_est) -> [Vpcc_dq_est]
  Current controller/1(Udq_ref1) -> [Udq_ref]
  [wt_ref] -> Subsystem3/2(wt)
  dq-abc/1(Uinv_ref1) -> [Uinv_ref]
  [wt_ref] -> dq-abc/2(wt)
  Iinv/1 -> Subsystem3/1(IL_abc)
  PWM/3(PWM3) -> PWM3/1
  Subsystem3/1(IL_dq_est) -> [I_Ldq_est]
  [wt_ref] -> Subsystem4/2(wt)
  PWM/1(PWM1) -> PWM1/1
  PWM/5(PWM5) -> PWM5/1
  PWM/6(PWM2) -> PWM2/1
  PWM/2("PWM4 ") -> "PWM4 "/1
  [Udq_ref] -> dq-abc/1(Udq_ref)
  [Uinv_ref] -> PWM/2(Uinv_ref)
  [Ipcc_dq] -> Voltage controller/1(Ipcc_est)
  Voltage controller/1(ILdq_ref) -> [iLdq_ref]
  [Vpcc_dq_est] -> Voltage controller/2(Vpcc_est)
  [iLdq_ref] -> Current controller/3(I_Ldq_ref)
  [wt_ref] -> Subsystem1/2(wt)
  Subsystem1/1(Uc_dq_est) -> [Ipcc_dq]
  Vpcc/1 -> [Vpcc]
  Ipcc/1 -> [Ipcc]
  [Vpcc] -> Subsystem4/1(Uc_abc)
  [Ipcc] -> Subsystem1/1(Uc_abc)
  [Vd_ref] -> Voltage controller/3(Vpcc_d_ref)

== system FullModelAddANN_Final_ANN_revised/Power cal2 ==
  In1 : Inport
  In2 : Inport  Port=2
  Demux10 : Demux  Outputs=3
  Demux11 : Demux  Outputs=3
  Subsystem8 : Subsystem
  Subsystem9 : Subsystem
  p3 : Subsystem
  q3 : Subsystem
  deltay1 : Outport
  deltay2 : Outport  Port=2
  wires:
  In1/1 -> Demux11/1
  In2/1 -> Demux10/1
  q3/1(deltay2) -> deltay2/1
  Demux10/1 -> Subsystem8/1(xa)
  Demux11/2 -> Subsystem9/2(xb)
  Demux11/1 -> Subsystem9/1(xa)
  Subsystem9/2(xbeta) -> q3/2(Beta), p3/2(Beta)
  p3/1(deltay1) -> deltay1/1
  Demux10/3 -> Subsystem8/3(xc)
  Subsystem9/1(xalpha) -> q3/1(Alpha), p3/1(Alpha)
  Demux10/2 -> Subsystem8/2(xb)
  Subsystem8/2(xbeta) -> q3/4(xbeta), p3/4(xbeta)
  Demux11/3 -> Subsystem9/3(xc)
  Subsystem8/1(xalpha) -> q3/3(xalpha), p3/3(xalpha)

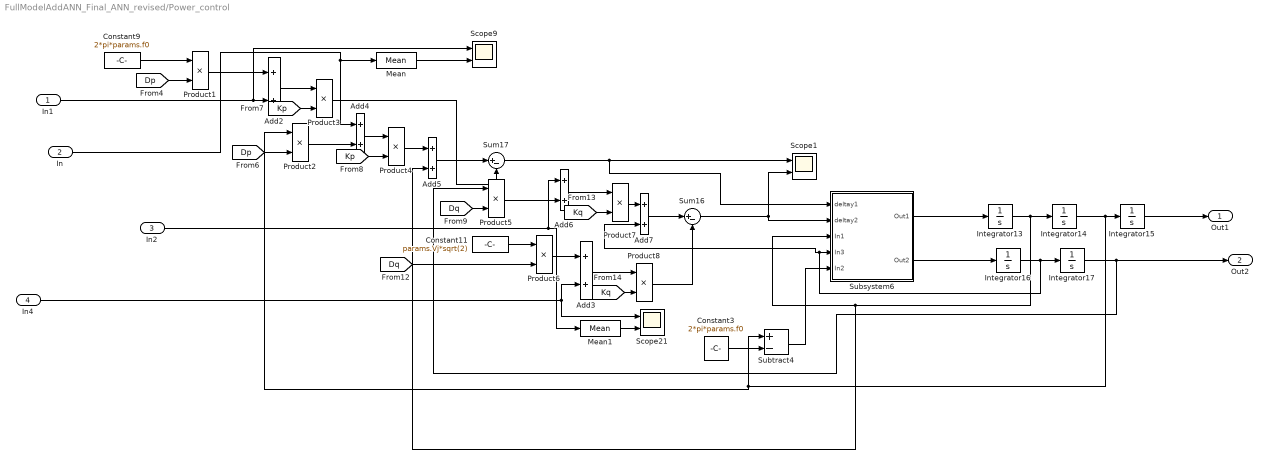
== system FullModelAddANN_Final_ANN_revised/Power_control ==
  In1 : Inport
  In : Inport  Port=2
  In2 : Inport  Port=3
  In4 : Inport  Port=4
  Add{2..7} (6 alike) : Sum
  Constant11 : Constant  Value=params.Vj*sqrt(2)
  Constant3 : Constant  Value=2*pi*params.f0
  Constant9 : Constant  Value=2*pi*params.f0
  Integrator13 : Integrator
  Integrator14 : Integrator  InitialCondition=2*pi*params.f0
  Integrator15 : Integrator  InitialCondition=0.034393045493197
  Integrator16 : Integrator
  Integrator17 : Integrator  InitialCondition=110.742
  Mean : spsMeanLib/Mean  Freq=60  Vinit=0  Ts=0
  Mean1 : spsMeanLib/Mean  Freq=60  Vinit=0  Ts=0
  Product{1..8} (8 alike) : Product
  Scope1 : Scope  NumInputPorts=2
  Scope21 : Scope  NumInputPorts=2
  Scope9 : Scope  NumInputPorts=2
  Subsystem6 : Subsystem
  Subtract4 : Sum  Inputs=+-
  Sum16 : Sum  Inputs=|+-
  Sum17 : Sum  Inputs=|+-
  Out1 : Outport
  Out2 : Outport  Port=2
  wires:
  Add6/1 -> Product7/1
  Integrator13/1 -> Integrator14/1, Subsystem6/3(In1), Add5/2
  Add2/1 -> Product3/1
  Product7/1 -> Add7/1
  Subtract4/1 -> Subsystem6/5(In2)
  Product4/1 -> Add5/1
  [Kp] -> Product3/2
  [Kq] -> Product8/2
  Subsystem6/2(Out2) -> Integrator16/1
  [Dp] -> Product1/2
  Sum16/1 -> Subsystem6/2(deltay2), Scope1/2
  In1/1 -> Scope9/1, Add2/2
  Mean/1 -> Scope9/2
  Sum17/1 -> Scope1/1, Subsystem6/1(deltay1)
  Constant11/1 -> Product6/1
  In2/1 -> Add6/1, Mean1/1
  [Kq] -> Product7/2
  [Kp] -> Product4/2
  Integrator14/1 -> Integrator15/1, Subtract4/1, Product2/1
  Mean1/1 -> Scope21/2
  Product3/1 -> Sum17/2
  Integrator17/1 -> Out2/1, Product5/1
  Subsystem6/1(Out1) -> Integrator13/1
  Add5/1 -> Sum17/1
  [Dq] -> Product5/2
  Add7/1 -> Sum16/1
  Product6/1 -> Add3/1
  In/1 -> Add4/1, Mean/1
  Add3/1 -> Product8/1
  Integrator16/1 -> Integrator17/1, Add7/2, Subsystem6/4(In3)
  Constant9/1 -> Product1/1
  Product5/1 -> Add6/2
  Product1/1 -> Add2/1
  Constant3/1 -> Subtract4/2
  Add4/1 -> Product4/1
  In4/1 -> Add3/2, Scope21/1
  [Dp] -> Product2/2
  [Dq] -> Product6/2
  Product8/1 -> Sum16/2
  Product2/1 -> Add4/2
  Integrator15/1 -> Out1/1

== system FullModelAddANN_Final_ANN_revised/Feed-Forward Neural Network2/Layer 1 ==
  "p{1}" : Inport  PortDimensions=200
      mask Display: e = 0.06;c1 = [120 230 180]/255;c2 = ([120 230 180]+0)/(256+128);c3 = ([120 230 180]+128)/(256+128);patch([0 1 1 0],[0 0 1 1],c1);patch([0 1 1 1-e 1-e 0+e],[0 0 1 1-e 0+e 0+e],c2);patch([0 0 1 1-e 0+e 0+e],[0 1 1 1-e 1-e 0+e],c3);plot([0 1 1 0 0],[0 0 1 1 0]);
  Delays 1 : Subsystem
      mask Display: e = 0.06;c1 = [120 150 230]/255;c2 = ([120 150 230]+0)/383;c3 = ([120 150 230]+128)/383;patch([0 1 1 0],[0 0 1 1],c1);patch([0 1 1 1-e 1-e 0+e],[0 0 1 1-e 0+e 0+e],c2);patch([0 0 1 1-e 0+e 0+e],[0 1 1 1-e 1-e 0+e],c3);plot([0 1 1 0 0],[0 0 1 1 0]);disp('0');
  "IW{1,1}" : Subsystem
      mask Display: e = 0.06;c1 = [120 150 230]/255;c2 = ([120 150 230]+0)/383;c3 = ([120 150 230]+128)/383;patch([0 1 1 0],[0 0 1 1],c1);patch([0 1 1 1-e 1-e 0+e],[0 0 1 1-e 0+e 0+e],c2);patch([0 0 1 1-e 0+e 0+e],[0 1 1 1-e 1-e 0+e],c3);plot([0 1 1 0 0],[0 0 1 1 0]);disp('W');
  "b{1}" : Constant  Value=[-0.1648415258202241273632893125977716408669948577880859375;-0.10005344841742809525175772478178259916603565216064453125;0.028394871693906774401394699225420481525361537933349609375;0.02039400079960096423548066013609059154987335205078125;-0.060644076225968825133438855345957563258707523345947265625;0.053394434198200661778610509600184741429984569549560546875;-0.030097290791324338155021678176126442849636077880859375;-0.2415236212881204658220468672880087979137897491455078125;0.0766402193814612331390634381023119203746318817138671875;-0.07175144906617451912023142313046264462172985076904296875;-0.026482277291088616999470417567863478325307369232177734375;0.07546916990557060722633053728714003227651119232177734375;0.068306338578225211932704041828401386737823486328125;-0.1890424898657833419068907687687897123396396636962890625;0.1335990029383468946644342167928698472678661346435546875;-0.1587399286170546874874531795285292901098728179931640625]
      mask Display: e = 0.06;c1 = [120 150 230]/255;c2 = ([120 150 230]+0)/383;c3 = ([120 150 230]+128)/383;patch([0 1 1 0],[0 0 1 1],c1);patch([0 1 1 1-e 1-e 0+e],[0 0 1 1-e 0+e 0+e],c2);patch([0 0 1 1-e 0+e 0+e],[0 1 1 1-e 1-e 0+e],c3);plot([0 1 1 0 0],[0 0 1 1 0]);disp('b');
  netsum : Sum  Inputs=2  InputSameDT=on  SaturateOnIntegerOverflow=on  OutDataTypeStr=Inherit: Same as first input
      mask Display: e = 0.06;c1 = [120 150 230]/255;c2 = ([120 150 230]+0)/383;c3 = ([120 150 230]+128)/383;patch([0 1 1 0],[0 0 1 1],c1);patch([0 1 1 1-e 1-e 0+e],[0 0 1 1-e 0+e 0+e],c2);patch([0 0 1 1-e 0+e 0+e],[0 1 1 1-e 1-e 0+e],c3);plot([0 1 1 0 0],[0 0 1 1 0]);disp('+');
  tansig : neural/Transfer Functions/tansig
  "a{1}" : Outport  InitialOutput=[0;0;0;0;0;0;0;0;0;0;0;0;0;0;0;0]
      mask Display: e = 0.06;c1 = [120 230 180]/255;c2 = ([120 230 180]+0)/(256+128);c3 = ([120 230 180]+128)/(256+128);patch([0 1 1 0],[0 0 1 1],c1);patch([0 1 1 1-e 1-e 0+e],[0 0 1 1-e 0+e 0+e],c2);patch([0 0 1 1-e 0+e 0+e],[0 1 1 1-e 1-e 0+e],c3);plot([0 1 1 0 0],[0 0 1 1 0]);
  wires:
  "p{1}"/1 -> Delays 1/1("p{1}")
  Delays 1/1("pd{1,1}") -> "IW{1,1}"/1("pd{1,1}")
  "IW{1,1}"/1("iz{1,1}") -> netsum/1
  "b{1}"/1 -> netsum/2
  netsum/1 -> tansig/1
  tansig/1 -> "a{1}"/1

== system FullModelAddANN_Final_ANN_revised/Feed-Forward Neural Network2/Layer 2 ==
  "a{1} " : Inport  PortDimensions=16
      mask Display: e = 0.06;c1 = [120 230 180]/255;c2 = ([120 230 180]+0)/(256+128);c3 = ([120 230 180]+128)/(256+128);patch([0 1 1 0],[0 0 1 1],c1);patch([0 1 1 1-e 1-e 0+e],[0 0 1 1-e 0+e 0+e],c2);patch([0 0 1 1-e 0+e 0+e],[0 1 1 1-e 1-e 0+e],c3);plot([0 1 1 0 0],[0 0 1 1 0]);
  Delays 1 : Subsystem
      mask Display: e = 0.06;c1 = [120 150 230]/255;c2 = ([120 150 230]+0)/383;c3 = ([120 150 230]+128)/383;patch([0 1 1 0],[0 0 1 1],c1);patch([0 1 1 1-e 1-e 0+e],[0 0 1 1-e 0+e 0+e],c2);patch([0 0 1 1-e 0+e 0+e],[0 1 1 1-e 1-e 0+e],c3);plot([0 1 1 0 0],[0 0 1 1 0]);disp('0');
  "LW{2,1}" : Subsystem
      mask Display: e = 0.06;c1 = [120 150 230]/255;c2 = ([120 150 230]+0)/383;c3 = ([120 150 230]+128)/383;patch([0 1 1 0],[0 0 1 1],c1);patch([0 1 1 1-e 1-e 0+e],[0 0 1 1-e 0+e 0+e],c2);patch([0 0 1 1-e 0+e 0+e],[0 1 1 1-e 1-e 0+e],c3);plot([0 1 1 0 0],[0 0 1 1 0]);disp('W');
  "b{2}" : Constant  Value=[-0.1489969950350367167146714564296416938304901123046875;0.361412922966195093721353259752504527568817138671875]
      mask Display: e = 0.06;c1 = [120 150 230]/255;c2 = ([120 150 230]+0)/383;c3 = ([120 150 230]+128)/383;patch([0 1 1 0],[0 0 1 1],c1);patch([0 1 1 1-e 1-e 0+e],[0 0 1 1-e 0+e 0+e],c2);patch([0 0 1 1-e 0+e 0+e],[0 1 1 1-e 1-e 0+e],c3);plot([0 1 1 0 0],[0 0 1 1 0]);disp('b');
  netsum : Sum  Inputs=2  InputSameDT=on  SaturateOnIntegerOverflow=on  OutDataTypeStr=Inherit: Same as first input
      mask Display: e = 0.06;c1 = [120 150 230]/255;c2 = ([120 150 230]+0)/383;c3 = ([120 150 230]+128)/383;patch([0 1 1 0],[0 0 1 1],c1);patch([0 1 1 1-e 1-e 0+e],[0 0 1 1-e 0+e 0+e],c2);patch([0 0 1 1-e 0+e 0+e],[0 1 1 1-e 1-e 0+e],c3);plot([0 1 1 0 0],[0 0 1 1 0]);disp('+');
  purelin : neural/Transfer Functions/purelin
  "a{2}" : Outport  InitialOutput=[0;0]
      mask Display: e = 0.06;c1 = [120 230 180]/255;c2 = ([120 230 180]+0)/(256+128);c3 = ([120 230 180]+128)/(256+128);patch([0 1 1 0],[0 0 1 1],c1);patch([0 1 1 1-e 1-e 0+e],[0 0 1 1-e 0+e 0+e],c2);patch([0 0 1 1-e 0+e 0+e],[0 1 1 1-e 1-e 0+e],c3);plot([0 1 1 0 0],[0 0 1 1 0]);
  wires:
  "a{1} "/1 -> Delays 1/1("p{2}")
  Delays 1/1("pd{2,1}") -> "LW{2,1}"/1("ad{2,1}")
  "LW{2,1}"/1("lz{2,1}") -> netsum/1
  "b{2}"/1 -> netsum/2
  netsum/1 -> purelin/1
  purelin/1 -> "a{2}"/1

== system FullModelAddANN_Final_ANN_revised/Feed-Forward Neural Network2/Process Input 1 ==
  x : Inport  PortDimensions=200
      mask Display: e = 0.06;c1 = [120 230 180]/255;c2 = ([120 230 180]+0)/(256+128);c3 = ([120 230 180]+128)/(256+128);patch([0 1 1 0],[0 0 1 1],c1);patch([0 1 1 1-e 1-e 0+e],[0 0 1 1-e 0+e 0+e],c2);patch([0 0 1 1-e 0+e 0+e],[0 1 1 1-e 1-e 0+e],c3);plot([0 1 1 0 0],[0 0 1 1 0]);
  mapminmax : neural/Processing Functions/mapminmax  xmin=[-14.3126999999999995338839653414;-2.92818999999999984851228873595;6.10846999999999962227548166993;20.4104999999999989768184605055;34.193399999999996907718013972;50.4232000000000013528733688872;66.110600000000005138645065017;78.9706999999999936790118226781;92.1013999999999981582732289098;93.2733999999999952024154481478;87.8075000000000045474735088646;81.8979999999999961346475174651;73.7858999999999980445863911882;68.173100000000005138645065017;66.5818000000000012050804798491;60.2032999999999987039700499736;52.0970999999999975216269376688;50.8479000000000027625901566353;42.8900999999999967826624924783;34.0756999999999976580511429347;30.2942000000000000170530256582;23.2284000000000006025402399246;17.3092000000000005854872142663;9.23129999999999917292825557524;9.91133999999999915075932221953;2.22879000000000004888534022029;-7.61038000000000014466650100076;-12.7484999999999999431565811392;-24.8626000000000004774847184308;-33.0225999999999970668795867823;-37.1724000000000032173375075217;-44.5686999999999997612576407846;-50.3708999999999988972376741003;-56.8751999999999995338839653414;-62.6968000000000031946001399774;-69.4508000000000009777068044059;-74.5177999999999940428097033873;-80.1586999999999960664354148321;-83.5424000000000006593836587854;-84.9556000000000040017766878009;-87.9736000000000046838977141306;-91.853099999999997749000613112;-92.345100000000002182787284255;-92.6796999999999968622432788834;-99.3796999999999997044142219238;-103.677000000000006707523425575;-104.948999999999998067323758733;-110.796999999999997044142219238;-106.367999999999994997779140249;-109.829999999999998294697434176;-110.558999999999997498889570124;-109.942999999999997839950083289;-107.789000000000001477928890381;-108.227999999999994429344951641;-111.843999999999994088284438476;-108.635000000000005115907697473;-107.332999999999998408384271897;-112.769000000000005456968210638;-116.650000000000005684341886081;-128.050000000000011368683772162;-133.522999999999996134647517465;-140.888000000000005229594535194;-148.270000000000010231815394945;-156.43600000000000704858393874;-163.98199999999999931787897367;-171.296999999999997044142219238;-174.342999999999989313437254168;-176.633000000000009777068044059;-178.069999999999993178789736703;-178.961999999999989086063578725;-179.669000000000011141310096718;-184.498999999999995225152815692;-187.042000000000001591615728103;-187.033999999999991814547684044;-186.116000000000013869794202037;-187.995000000000004547473508865;-183.979999999999989768184605055;-182.060000000000002273736754432;-179.549000000000006593836587854;-178.843999999999994088284438476;-174.376000000000004774847184308;-173.641999999999995907273842022;-174.37799999999998590283212252;-173.592000000000012960299500264;-170.056000000000011596057447605;-161.650000000000005684341886081;-152.899000000000000909494701773;-141.338999999999998635757947341;-129.032000000000010686562745832;-115.799000000000006593836587854;-102.715999999999993974597600754;-88.3242000000000047066350816749;-76.417199999999994020072335843;-62.9399000000000015120349416975;-52.5930000000000035242919693701;-40.3836999999999974875208863523;-33.0645999999999986584953148849;-28.3279999999999994031441019615;-23.4516999999999988801846484421;-21.7592999999999996418864611769;-8.96842999999999967997155181365;-8.94142000000000081172402133234;-9.04396999999999984254372975556;-9.0359499999999997044142219238;-8.80085000000000050590642786119;-8.37179000000000073100636654999;-7.74662000000000006139089236967;-6.92257999999999995566213328857;-5.87485999999999997100985638099;-4.74976999999999982549070409732;-3.70647999999999999687361196266;-2.50839999999999996305177774047;-1.37159999999999993036681189551;-0.546263999999999971812769672397;0.352642000000000011006306976924;1.52173000000000002707167823246;2.70387000000000021771029423689;3.66676000000000001932676241267;4.31484000000000023078428057488;4.85635999999999956600049699773;5.38818999999999981298515194794;6.24335000000000039932501749718 ...(+2537 chars)]  xmax=[110.751000000000004774847184308;111.968999999999994088284438476;110.581000000000003069544618484;111.900999999999996248334355187;110.879000000000004888534022029;109.5139999999999957935870043;108.072000000000002728484105319;112.727999999999994429344951641;116.915000000000006252776074689;126.253000000000000113686837722;133.5279999999999915871740086;140.966000000000008185452315956;147.711999999999989086063578725;156.89300000000000068212102633;163.828000000000002955857780762;170.586999999999989086063578725;175.444999999999993178789736703;175.879999999999995452526491135;177.181000000000011596057447605;179.770999999999986584953148849;185.185000000000002273736754432;185.889999999999986357579473406;184.932999999999992724042385817;186.064999999999997726263245568;185.510999999999995679900166579;183.180000000000006821210263297;183.29300000000000636646291241;182.115000000000009094947017729;179.734000000000008867573342286;177.973999999999989540810929611;176.131000000000000227373675443;175.824999999999988631316227838;173.01800000000000068212102633;170.937999999999988176568876952;169.888000000000005229594535194;160.532999999999987039700499736;155.93600000000000704858393874;143.931000000000011596057447605;130.037000000000006139089236967;117.489000000000004320099833421;105.33199999999999363353708759;88.7804000000000002046363078989;74.479699999999994020072335843;63.1747999999999976239450916182;52.6728000000000022851054382045;43.0095000000000027284841053188;33.8121999999999971464603731874;27.3789000000000015688783605583;22.683499999999998664179656771;21.5057000000000009265477274312;14.0518999999999998351540853037;4.86477000000000003865352482535;-6.09895000000000031548097467748;-17.5753999999999983572251949226;-32.9281000000000005911715561524;-49.7428999999999987835508363787;-64.7210000000000036379788070917;-78.334400000000002250999386888;-91.0614000000000061163518694229;-89.1077999999999974534148350358;-88.1247999999999933606886770576;-82.7978999999999984993337420747;-77.2025000000000005684341886081;-70.2156999999999982264853315428;-63.9776999999999986812326824293;-55.5390999999999976921571942512;-51.1319999999999978967935021501;-46.9172999999999973397279973142;-40.5180999999999968963493301999;-33.9275000000000019895196601283;-34.1165000000000020463630789891;-26.2178000000000004376943252282;-19.2653999999999996362021192908;-12.3146000000000004348521542852;-5.01944000000000034589220376802;-1.4204000000000001069366817319;3.55146000000000006124878382252;14.7215000000000006963318810449;20.2200999999999986300736054545;28.7895000000000003126388037344;36.2411999999999991928234521765;42.8667999999999977944753482006;49.5801999999999978285813995171;56.4909999999999996589394868352;61.5112999999999985334397933912;66.7223999999999932697392068803;72.0896999999999934516381472349;77.6791999999999944748196867295;81.9883999999999986130205797963;83.7926999999999964074959279969;87.4411999999999949295670376159;91.2070999999999969531927490607;96.4641000000000019554136088118;100.555000000000006821210263297;103.409999999999996589394868352;106.046999999999997044142219238;105.052000000000006707523425575;104.85699999999999931787897367;105.435000000000002273736754432;107.974999999999994315658113919;104.296000000000006480149750132;102.911000000000001364242052659;101.132999999999995566213328857;99.0812999999999988176568876952;96.7026000000000038880898500793;93.9581000000000017280399333686;90.8442000000000007275957614183;87.2887000000000057298166211694;83.2707999999999941564965411089;78.907600000000002182787284255;74.254800000000003024069883395;69.1995000000000004547473508865;63.7882999999999995566213328857;57.9904999999999972715158946812;52.1182000000000016370904631913;46.107900000000000773070496507;39.8301000000000016143530956469;33.5949000000000026489033189137;27.4848999999999996646238287212;23.5473999999999996646238287212;20.1804999999999985504928190494;17.3689000000000000056843418861;14.8262000000000000454747350886;14.9801999999999999602096067974 ...(+2435 chars)]  ymin=-1  ymax=1
  p : Outport  PortDimensions=200
      mask Display: e = 0.06;c1 = [120 230 180]/255;c2 = ([120 230 180]+0)/(256+128);c3 = ([120 230 180]+128)/(256+128);patch([0 1 1 0],[0 0 1 1],c1);patch([0 1 1 1-e 1-e 0+e],[0 0 1 1-e 0+e 0+e],c2);patch([0 0 1 1-e 0+e 0+e],[0 1 1 1-e 1-e 0+e],c3);plot([0 1 1 0 0],[0 0 1 1 0]);
  wires:
  x/1 -> mapminmax/1
  mapminmax/1 -> p/1
